simulink model "abcd"  (R2020a)
settings: Solver=FixedStepAuto  StartTime=0.0  StopTime=1  RelTol=1e-3
libraries: powerlib x9, androiduilib x5, re_lib x1, powerlib_meascontrol x1
settings Model: Creator=kushalgoswami  LastModifiedBy=kushalgoswami
settings OptimizationCC: EnhancedBackFolding=on  PassReuseOutputArgsAs=Individual arguments  ZeroExternalMemoryAtStartup=off  ZeroInternalMemoryAtStartup=off  MaxStackSize=64  OptimizeBlockOrder=speed  DifferentSizesBufferReuse=on  OptimizationCustomize=off  EfficientTunableParamExpr=on
settings DebuggingCC: ParameterTunabilityLossMsg=error
settings HardwareCC: ProdBitPerPointer=32  ProdBitPerSizeT=32  ProdBitPerPtrDiffT=32  ProdLargestAtomicInteger=Long  ProdLargestAtomicFloat=Double  ProdWordSize=32  ProdHWDeviceType=ARM Compatible->ARM Cortex  UseEmbeddedCoderFeatures=off  UseSimulinkCoderFeatures=off
settings SFSimCC: MATLABDynamicMemAlloc=off
settings RTWCC: SystemTargetFile=ert.tlc  HardwareBoard=Android Device  TemplateMakefile=ert_default_tmf  RTWVerbose=off  Toolchain=Android SDK/NDK Tools
settings CodeAppCC: ForceParamTrailComments=on  IgnoreCustomStorageClasses=off  OperatorAnnotations=on  SimulinkDataObjDesc=on  SFDataObjDesc=on  InsertBlockDesc=on
settings ERTTargetCC: SupportNonInlinedSFcns=on

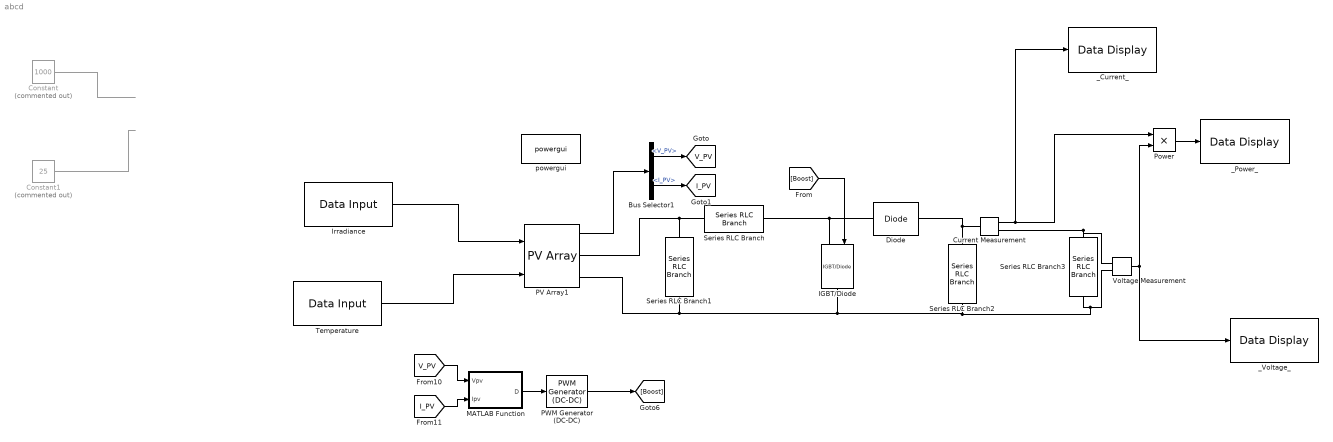
== system abcd ==
  Bus Selector1 : BusSelector  OutputSignals=V_PV,I_PV
  Constant : Constant  Commented=on  Value=1000
  Constant1 : Constant  Commented=on  Value=25
  Current Measurement : powerlib/Measurements/Current Measurement  PhasorSimulation=off  OutputType=Complex  PSBequivalent=0
  Diode : powerlib/Power Electronics/Diode  Ron=0.001  Lon=0  Vf=0.8  IC=0  UseSnubber=0  Rs=500  Cs=250e-9  Measurements=off
  IGBT/Diode : powerlib/Power Electronics/IGBT//Diode  Ron=1e-3  Rs=1e5  Cs=inf  Measurements=off
  Irradiance : androiduilib/Data Input  isCharVector=off  Value=1000  CharVector=Hello World  OutputDataType=int32  maxCharVectorSize=100  DataInputId=abcd/Irradiance  SampleTime=0.1
      settings: SourceProductBaseCode=ANDROID
  MATLAB Function : MATLAB Function  TreatAsAtomicUnit=on
  PV Array1 : re_lib/Solar/PV Array  Npar=1  Nser=1  PlotType=array @ 1000 W/m2 & specified temperatures  S_vec="[ 1000  500  100 ]"  Temp_C_vec="[ 45 25  ]"  ModuleName=1Soltech 1STH-250-WH  PlotWhenSelected=off  Pm=250.205  Ncell=60  Voc=37.3  Isc=8.66  Vm=30.7  Im=8.15  beta_Voc_pc=-0.36901  alpha_Isc_pc=0.086998  beta_Voc=-0.13764  alpha_Isc=0.007534  IL=8.7106  I0=4.1601e-10  nI=1.019  Rsh=224.1886  Rs=0.23724  RobustModel=off  RobustCellTemperature=25  BAL=on  Tc=1e-6  Tfilter=5e-5
  PWM Generator (DC-DC) : powerlib_meascontrol/Pulse & Signal Generators/PWM Generator (DC-DC)  Fsw=5000  Ts=10e-6
  Power : Product
  Series RLC Branch : powerlib/Elements/Series RLC Branch  LConnTagsString=__new0  RConnTagsString=__new0  BranchType=L  Resistance=0.1  Inductance=5e-3  SetiL0=off  InitialCurrent=0  Capacitance=1e-6  Setx0=off  InitialVoltage=0  Measurements=None
  Series RLC Branch1 : powerlib/Elements/Series RLC Branch  LConnTagsString=__new0  RConnTagsString=__new0  BranchType=C  Resistance=1e-4  Inductance=1e-3  SetiL0=off  InitialCurrent=0  Capacitance=100e-6  Setx0=off  InitialVoltage=0  Measurements=None
  Series RLC Branch2 : powerlib/Elements/Series RLC Branch  LConnTagsString=__new0  RConnTagsString=__new0  BranchType=C  Resistance=1e-4  Inductance=1e-3  SetiL0=off  InitialCurrent=0  Capacitance=3300e-6  Setx0=off  InitialVoltage=0  Measurements=None
  Series RLC Branch3 : powerlib/Elements/Series RLC Branch  LConnTagsString=__new0  RConnTagsString=__new0  BranchType=R  Resistance=10  Inductance=1e-3  SetiL0=off  InitialCurrent=0  Capacitance=3300e-6  Setx0=off  InitialVoltage=0  Measurements=None
  Temperature : androiduilib/Data Input  isCharVector=off  Value=25  CharVector=Hello World  OutputDataType=int32  maxCharVectorSize=100  DataInputId=abcd/Temperature  SampleTime=0.1
      settings: SourceProductBaseCode=ANDROID
  Voltage Measurement : powerlib/Measurements/Voltage Measurement  PhasorSimulation=off  OutputType=Complex  PSBequivalent=0
  _Current_ : androiduilib/Data Display  DataDisplayId=abcd/_Current_  Format=Float  Precision=6  SimulateUsing=Code generation  blockPlatform=Android
      settings: SourceProductBaseCode=ANDROID
  _Power_ : androiduilib/Data Display  DataDisplayId=abcd/_Power_  Format=Float  Precision=6  SimulateUsing=Code generation  blockPlatform=Android
      settings: SourceProductBaseCode=ANDROID
  _Voltage_ : androiduilib/Data Display  DataDisplayId=abcd/_Voltage_  Format=Float  Precision=6  SimulateUsing=Code generation  blockPlatform=Android
      settings: SourceProductBaseCode=ANDROID
  powergui : powerlib/powergui  Priority=1  SimulationMode=Discrete  SampleTime=50e-6  frequency=60  Iterations=50  frequencyindice=0  Pbase=100e6  ErrMax=1e-4  UnitsV=kV  UnitsW=MW  buscounter=0  FunctionMessages=off  echomessages=off  EnableUseOfTLC=off  CurrentSourceSwitches=off  DisableSnubberDevices=off  DisableRonSwitches=off  DisableVfSwitches=off  DisplayEquations=off  AutomaticDiscreteSolvers=off  SolverType=Tustin/Backward Euler (TBE)  Interpol=off  ExternalGateDelay=off  methode=off  Ts=100  x0status=blocks  SPID=on  SwTol=0  HookPort=off  NonlinearTolerance=1e-4  nMaxIteration=100  ContinueOnMaxIteration=off  RestoreLinks=warning  ResistiveCurrentMeasurement=off  Frange=[0:2:500]  Ylog=off  Xlog=on  ShowGrid=off  save=off  variable=ZData  structure=0  ZoomFFT=off  StartTime=0.0  cycles=1  DisplayStyle=1  fundamental=60  FreqAxis=off  MaxFrequency=1000  frequencyindicesteady=1  RmsSteady=1  display=off
  tag scope: I_PV=global, V_PV=global
  wires:
  Power/1 -> _Power_/1
  [I_PV] -> MATLAB Function/2(Ipv)
  Voltage Measurement/1 -> Power/2, _Voltage_/1
  [Boost] -> IGBT/Diode/1
  Current Measurement/1 -> _Current_/1, Power/1
  Bus Selector1/2 -> [I_PV]  "<I_PV>"
  PV Array1/1 -> Bus Selector1/1
  Bus Selector1/1 -> [V_PV]  "<V_PV>"
  PWM Generator (DC-DC)/1 -> [Boost]
  MATLAB Function/1(D) -> PWM Generator (DC-DC)/1
  [V_PV] -> MATLAB Function/1(Vpv)
  Constant1/1 -> ?
  Constant/1 -> ?
  Irradiance/1 -> PV Array1/1
  Temperature/1 -> PV Array1/2
  connections:
  Diode/RConn1 -- Current Measurement/LConn1 -- Series RLC Branch2/LConn1
  Series RLC Branch1/RConn1 -- IGBT/Diode/RConn1 -- Voltage Measurement/LConn2 -- Series RLC Branch3/RConn1 -- Series RLC Branch2/RConn1 -- PV Array1/RConn2
  Series RLC Branch/RConn1 -- Diode/LConn1 -- IGBT/Diode/LConn1
  Voltage Measurement/LConn1 -- Current Measurement/RConn1 -- Series RLC Branch3/LConn1
  PV Array1/RConn1 -- Series RLC Branch1/LConn1 -- Series RLC Branch/LConn1

== matlab function abcd/MATLAB Function ==
  data: Vpv input; D output; Ipv input
function D = PO(Vpv,Ipv)

Dinit=0.42;
Dmax=0.8;
Dmin=0.08;
deltaD=0.000005;

persistent Dprev Pprev Vprev

if isempty(Vprev)
    Vprev=0;
    Dprev=Dinit;
    Pprev=0;
end

deltaD=125e-6;

Ppv=Vpv*Ipv;

if (Ppv-Pprev)~=0
    if (Ppv-Pprev)>0
        if (Vpv-Vprev)>0
            D=Dprev-deltaD;
        else
            D=Dprev+deltaD;
        end
    else
        if (Vpv-Vprev)>0
            D=Dprev+deltaD;
        else
            D=Dprev-deltaD;
        end
    end
else
    D=Dprev;
end

if D>=Dmax | D<=Dmin
    D=Dprev;
end
Dprev=D;
Vprev=Vpv;
Pprev=Ppv;
